simulink model "geoSub"  (R2022b)
settings: Solver=VariableStepAuto  StartTime=0.0  StopTime=10.0  RelTol=1e-3
libraries: ros2lib x1
settings Model: Creator=System-10  LastModifiedBy=System-10

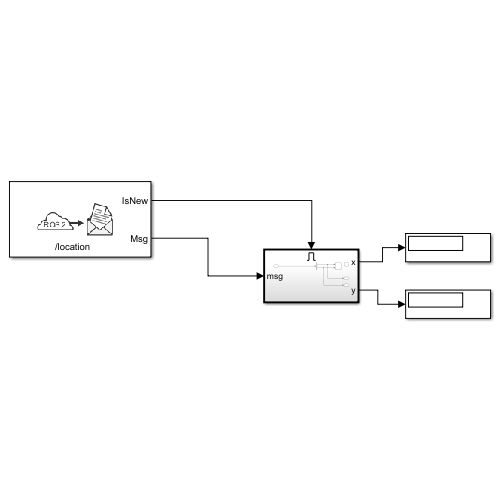
[thumbnail: Simulink's stored preview of the top-level diagram]
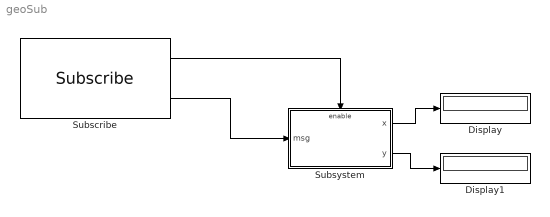
== system geoSub ==
  Display : Display
  Display1 : Display
  Subscribe : ros2lib/Subscribe  topicSource=Specify your own  topic=/location  messageType=geometry_msgs/Point  sampleTime=Ts  QOSHistory=Keep last  QOSDepth=1  QOSReliability=Reliable  QOSDurability=Volatile
      settings: LibrarySourceBlock=roslib/ROS 2/Subscribe
  Subsystem : Subsystem
  wires:
  Subscribe/2 -> Subsystem/1(msg)
  Subsystem/1(x) -> Display/1
  Subsystem/2(y) -> Display1/1
  Subscribe/1 -> Subsystem/Enable

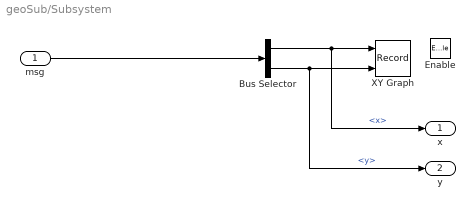
== system geoSub/Subsystem ==
  msg : Inport
  Enable : EnablePort
  Bus Selector : BusSelector  OutputSignals=x,y
  XY Graph : Record  FileSettingsInternal="{\"entries\":[{\"content\":{\"excelSettings\":{\"content\":{},\"type\":\"Streamout.ExcelSettings\"}},\"type\":\"Streamout.FileSettingStorage\",\"uuid\":\"132e89df-0712-48a6-a386-eeb90432fbcf\"}],\"packageUris\":[\"http://schema.mathworks.com/mf0/streamout_blocks/R2020a\"],\"version\":\"1.0\"}"  Layout=[1 1]  SignalsInternal="{\"entries\":[{\"content\":{\"signals\":[{\"content\":{\"blockPath\":[\"geoSub/Subsystem/XY Graph\"],\"channel\":[],\"dimensions\":[1],\"domain\":\"geoSub/Subsystem/XY Graph\",\"lineColor\":\"#ff6929\",\"plots\":[],\"port\":1,\"sid\":[\"\"],\"signalID\":1642,\"signalName\":\"<x>\"},\"type\":\"RecordBlkView.Signal\",\"uuid\":\"3ac900ff-c0fe-4014-972c-ba076dca31cd\"},{\"content\":{\"blockPath\":[\"geoSub/Subsystem/XY Graph\"],\"channel\":[],\"dimensions\":[1],\"domain\":\"geoSub/Subsystem/XY Graph\",\"lineColor\":\"#b746ff\",\"plots\":[],\"port\":2,\"sid\":[\"\"],\"signalID\":1646,\"signalName\":\"<y>\"},\"type\":\"RecordBlkView.Signal\",\"uuid\":\"52e0db14-ddc7-4365-80d7-18bb62ef9dc7\"}]},\"type\":\"RecordBlkView.InputSignals\",\"uuid\":\"df974989-76c3-435f-b81e-a627231461e9\"}],\"packageUris\":[\"http://schema.mathworks.com/mf0/streamout_blocks/R2020a\"],\"version\":\"1.0\"}"  VisualizationBindings="{\"xyplotplugin\":{\"info\":[{\"series\":[],\"subplotID\":1}]}}"  CompatibilityTag=XY
  x : Outport
  y : Outport  Port=2
  wires:
  msg/1 -> Bus Selector/1
  Bus Selector/1 -> XY Graph/1, x/1  "<x>"
  Bus Selector/2 -> XY Graph/2, y/1  "<y>"
